simulink model "angularOnlinePIDTuningR2019a"  (R2019a)
settings: Solver=FixedStepAuto  StartTime=0.0  StopTime=100  RelTol=1e-3
model workspace (MAT data in the model file):
  p = [-7.82997288351e-05; 0.181210895977; -0.072497134344; 0.000486358314052; 0.0361674637937]
libraries: arduinolib x7, simulink x3, slctrlblks x1, simulink_extras x1
settings Model: SimulationMode=external  ExtModeTrigDuration=2  Creator=The MathWorks, Inc.  LastModifiedBy=manh
settings DataIOCC: ReturnWorkspaceOutputs=off
settings OptimizationCC: PassReuseOutputArgsAs=Individual arguments  MaxStackSize=64
settings DebuggingCC: ParameterPrecisionLossMsg=none  ParameterTunabilityLossMsg=error  ArithmeticOperatorsInVariantConditions=warning
settings HardwareCC: ProdBitPerInt=16  ProdBitPerPointer=16  ProdBitPerSizeT=16  ProdBitPerPtrDiffT=16  ProdLargestAtomicFloat=None  ProdWordSize=8  ProdHWDeviceType=Atmel->AVR
settings SFSimCC: SimUseLocalCustomCode=off  MATLABDynamicMemAlloc=off
settings RTWCC: SystemTargetFile=ert.tlc  HardwareBoard=Arduino Mega 2560  TLCOptions=-aInlineSetEventsForThisBaseRateFcn=TLC_FALSE -aSuppressMultiTaskScheduler=TLC_FALSE -aRateBasedStepFcn=1  TemplateMakefile=ert_default_tmf  GenerateReport=on  RTWUseLocalCustomCode=off  Toolchain=Arduino AVR  BuildConfiguration=Faster Runs  IncludeHyperlinkInReport=on  LaunchReport=on  GenerateTraceInfo=on  GenerateTraceReport=on  GenerateTraceReportSl=on  GenerateTraceReportSf=on  GenerateTraceReportEml=on
settings CodeAppCC: ForceParamTrailComments=on  IgnoreCustomStorageClasses=off  OperatorAnnotations=on  SimulinkDataObjDesc=on  SFDataObjDesc=on  InsertBlockDesc=on
settings ERTTargetCC: SupportContinuousTime=on  SupportVariableSizeSignals=on

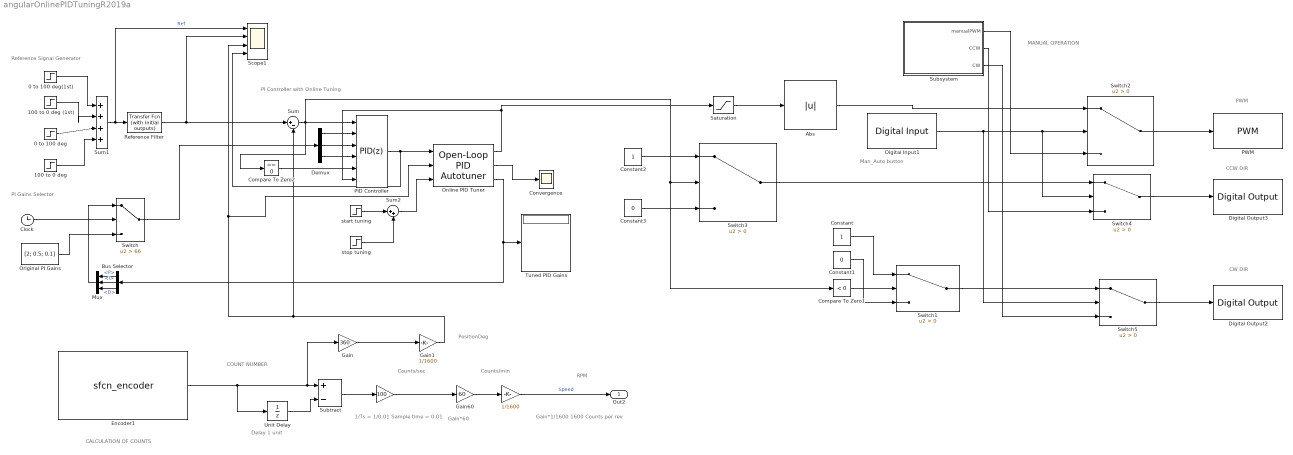
== system angularOnlinePIDTuningR2019a ==
  note: PI Gains Selector
  note: PI Controller with Online Tuning
  note: Reference Signal Generator
  note: COUNT NUMBER
  note: Gain*1/1600
      | 1600 Counts per rev
  note: Man_Auto button
  note: Counts/sec
  note: CW DIR
  note: CALCULATION OF COUNTS
  note: MANUAL OPERATION
  note: Delay 1 unit
  note: PWM
  note: Gain*60
  note: RPM
  note: Counts/min
  note: CCW DIR
  note: 1/Ts = 1/0.01
      | Sample time = 0.01
  note: PositionDeg
  " " : Gain  Gain=100  OutDataTypeStr=double
  " " : Gain  Gain=1/1600  OutDataTypeStr=double
  "0 to 100 deg " : Step  Time=60  After=100  SampleTime=0
  0 to 100 deg(1st) : Step  Time=2  After=100  SampleTime=0
  100 to 0 deg : Step  Time=80  After=-100  SampleTime=0
  100 to 0 deg (1st) : Step  Time=20  After=-100  SampleTime=0
  Abs : Abs
  Bus Selector : BusSelector  OutputSignals=P,I,D
  Clock : Clock
  Compare To Zero1 : simulink/Logic and Bit Operations/Compare To Zero  relop=<  OutDataTypeStr=boolean
  Compare To Zero2 : simulink/Logic and Bit Operations/Compare To Zero  relop===  OutDataTypeStr=boolean
  Constant : Constant
  Constant1 : Constant  Value=0
  Constant2 : Constant
  Constant3 : Constant  Value=0
  Convergence : Scope
  Demux : Demux  Outputs=3
  Digital Input1 : arduinolib/Digital Input  pinNumber=28  sampleTime=0.01  blockPlatform=arduino
      settings: SourceProductName=Simulink Support Package for Arduino Hardware
  Digital Output2 : arduinolib/Digital Output  pinNumber=38  blockPlatform=arduino
  Digital Output3 : arduinolib/Digital Output  pinNumber=36  blockPlatform=arduino
  Encoder1 : S-Function  InitFcn=try, set_param(gcb,'FunctionName','sfcn_encoder'), end  FunctionName=sfcn_encoder  Parameters=uint8(0),uint8(2),uint8(3)  SFunctionModules=sfcn_encoder_wrapper  SFunctionDeploymentMode=off  EnableBusSupport=off  mask(S-Function Builder){}
      mask init:
      | val = [[.9  0.75 0.75 1 1 .9 .9 1]',[1 1 0.75 0.75 .9 .9 1 .9]'];try , sys = get_param(gcb,'SfunBuilderFcnName');if isempty(sys), sys = get_param(gcb,'FunctionName'); end,catch, sys = get_param(gcb,'FunctionName'); end
      settings: CopyFcn=set_param(gcbh,'LinkStatus','none')  PreSaveFcn=try, set_param(gcb,'FunctionName','sfcn_encoder'), end  OpenFcn=sfunctionwizard(gcbh)
      mask Display: plot(val(:,1),val(:,2)),disp(sys), port_label('output',1,'pos')
  Gain : Gain  Gain=360  ParamDataTypeStr=double  OutDataTypeStr=double
  Gain1 : Gain  Gain=1/1600  ParamDataTypeStr=double  OutDataTypeStr=double
  Gain60 : Gain  Gain=60  OutDataTypeStr=double
  Mux : Mux  Inputs=3
  Online PID Tuner : slctrlblks/Open-Loop PID Autotuner  PIDType=PID  PIDForm=Parallel  TimeDomain=discrete-time  DiscreteTs=0.1  IntegratorFormula=Forward Euler  FilterFormula=Forward Euler  ContinuousTs=0.02  Bandwidth=2  UseExternalWC=off  TargetPM=60  UseExternalPM=off  UseExternalAchievedPM=off  AmpSine=0.1  UseExternalAmpSine=off  EstimateDCGain=on  AmpStep=0.1  UseExternalAmpStep=off  UseExternalFRD=off  UseExternalU0=off  UseExternalDCGain=off  NotDeployTuningModule=on  UsePLCCoder=off  BlockDataType=double  UseConnectedPID=on  blockpath=[]  tunedP=0  tunedI=0  tunedD=0  tunedN=100  tunedPM=0  EstimationWindowSize=4
      settings: SourceProductName=Simulink Control Design  SourceProductBaseCode=SD
  Original PI Gains : Constant  Value=[2; 0.5; 0.1]
  PID Controller : simulink/Continuous/PID Controller  Tag=PID1  Controller=PID  Form=Parallel  TimeDomain=Discrete-time  SampleTime=0.01  IntegratorMethod=Forward Euler  FilterMethod=Forward Euler  ControllerParametersSource=external  P=0.01  I=0.01  D=0  UseFilter=off  N=100  TunerSelectOption=Transfer Function Based (PID Tuner App)  ZeroCross=off  InitialConditionSource=internal  InitialConditionForIntegrator=0  InitialConditionForFilter=0  DifferentiatorICPrevScaledInput=0  ExternalReset=either  TrackingMode=on  Kt=1  LimitOutput=on  UpperSaturationLimit=255  LowerSaturationLimit=-255  LinearizeAsGain=off  AntiWindupMode=back-calculation  Kb=1  POutMin=[ ]  POutMax=[ ]  IOutMin=[ ]  IOutMax=[ ]  DOutMin=[ ]  DOutMax=[ ]  NOutMin=[ ]  NOutMax=[ ]  SumOutMin=[ ]  SumOutMax=[ ]  SaturationOutMin=[ ]  SaturationOutMax=[ ]  PParamMin=[ ]  PParamMax=[ ]  IParamMin=[ ]  IParamMax=[ ]  DParamMin=[ ]  DParamMax=[ ]  NParamMin=[ ]  NParamMax=[ ]  KbParamMin=[ ]  KbParamMax=[ ]  KtParamMin=[ ]  KtParamMax=[ ]  KbOutMin=[ ]  KbOutMax=[ ]  KtOutMin=[ ]  KtOutMax=[ ]  IntegratorOutMin=[ ]  IntegratorOutMax=[ ]  FilterOutMin=[ ]  FilterOutMax=[ ]  SumI1OutMin=[ ]  SumI1OutMax=[ ]  SumI2OutMin=[ ]  SumI2OutMax=[ ]  SumI3OutMin=[ ]  SumI3OutMax=[ ]  SumI4OutMin=[]  SumI4OutMax=[]  SumDOutMin=[ ]  SumDOutMax=[ ]  DifferentiatorOutMin=[]  DifferentiatorOutMax=[]  FilterDiffOutCoefMin=[]  FilterDiffOutCoefMax=[]  ReciprocalOutMin=[]  ReciprocalOutMax=[]  SumDenOutMin=[]  SumDenOutMax=[]  SumNumOutMin=[]  SumNumOutMax=[]  DivideOutMin=[]  DivideOutMax=[]  IntegratorContinuousStateAttributes=''  IntegratorStateMustResolveToSignalObject=off  IntegratorRTWStateStorageClass=Auto  FilterContinuousStateAttributes=''  FilterStateMustResolveToSignalObject=off  FilterRTWStateStorageClass=Auto  ParallelPVariant=ExternalParameters  IdealPVariant=Disabled  IVariant=ExternalParameters  DVariant=ExternalParameters  IntegratorVariant=Discrete  SatVariant=Enabled  AWVariant=BackCalculation  PCopyVariant=Disabled  TRVariant=Enabled  FdbkBlocksVariant=Forward  IdealPFdbkVariant=Disabled  SatFdbkVariant=Disabled  DerivativeFilterVariant=Differentiator  NVariant=Passthrough  NCopyVariant=Disabled_SignalSpec  FilterICVariant=InternalICsDifferentiator  IntegratorICVariant=InternalICs  ExternalResetVariant=ExternalReset  TRSumVariant=TrackingMode  SumFdbkVariant=Disabled  SumVariant=Sum_PID
  PWM : arduinolib/PWM  pinNumber=7  EnableInputFrequency=off  InitialFrequency=2000  InitialDutyCycle=0  NotificationType=None  blockPlatform=arduino
  Reference Filter : simulink_extras/Additional Linear/Transfer Fcn (with initial outputs)  N=[10]  D="[1  10]"  Y0=0  U0=0
  Saturation : Saturate  UpperLimit=255  LowerLimit=-255
  Scope1 : Scope  NumInputPorts=4
  Subsystem : Subsystem
  Subtract : Sum  Inputs=+-
  Sum : Sum  Inputs=|+-
  Sum1 : Sum  Inputs=|++++
  Sum2 : Sum  Inputs=|++
  Switch : Switch  Criteria=u2 > Threshold  Threshold=66
  Switch{1..5} (5 alike) : Switch  Criteria=u2 > Threshold
  Tuned PID Gains : Display
  Unit Delay : UnitDelay  SampleTime=-1  HasFrameUpgradeWarning=on
  start tuning : Step  Time=30  SampleTime=0
  stop tuning : Step  Time=65  After=-1  SampleTime=0
  Out2 : Outport  SignalName=speedRPM
  wires:
  Bus Selector/1 -> Mux/1  "<P>"
  100 to 0 deg/1 -> Sum1/4
  Original PI Gains/1 -> Switch/3
  Bus Selector/2 -> Mux/2  "<I>"
  Online PID Tuner/1 -> Saturation/1, PID Controller/6
  Online PID Tuner/3 -> Bus Selector/1, Tuned PID Gains/1
  Demux/1 -> PID Controller/2
  PID Controller/1 -> Scope1/4, Online PID Tuner/1
  Sum1/1 -> Scope1/1, Reference Filter/1  "Ref"
  Sum/1 -> Compare To Zero1/1, Switch3/2, PID Controller/1, Compare To Zero2/1
  Reference Filter/1 -> Sum/1, Scope1/2
  "0 to 100 deg "/1 -> Sum1/3
  Online PID Tuner/2 -> Convergence/1
  Demux/2 -> PID Controller/3
  Sum2/1 -> Online PID Tuner/3
  stop tuning/1 -> Sum2/2
  start tuning/1 -> Sum2/1
  100 to 0 deg (1st)/1 -> Sum1/2
  Switch/1 -> Demux/1
  Mux/1 -> Switch/1
  Gain1/1 -> Sum/2, Online PID Tuner/2, Scope1/3
  Switch3/1 -> Switch4/1
  " "/1 -> Out2/1  "Speed"
  Subsystem/2(CCW) -> Switch4/3
  Gain60/1 -> " "/1
  Gain/1 -> Gain1/1
  Switch2/1 -> PWM/1
  Switch1/1 -> Switch5/1
  Subsystem/3(CW) -> Switch5/3
  Constant/1 -> Switch1/1
  Saturation/1 -> Abs/1
  Abs/1 -> Switch2/1
  Constant1/1 -> Switch1/3
  Constant3/1 -> Switch3/3
  Constant2/1 -> Switch3/1
  " "/1 -> Gain60/1
  Unit Delay/1 -> Subtract/2
  Subsystem/1(manualPWM) -> Switch2/3
  Encoder1/1 -> Gain/1, Subtract/1, Unit Delay/1
  Switch4/1 -> Digital Output3/1
  Switch5/1 -> Digital Output2/1
  Subtract/1 -> " "/1
  Digital Input1/1 -> Switch2/2, Switch4/2, Switch5/2
  Clock/1 -> Switch/2
  0 to 100 deg(1st)/1 -> Sum1/1
  Compare To Zero1/1 -> Switch1/2
  Bus Selector/3 -> Mux/3  "<D>"
  Compare To Zero2/1 -> PID Controller/5
  Demux/3 -> PID Controller/4

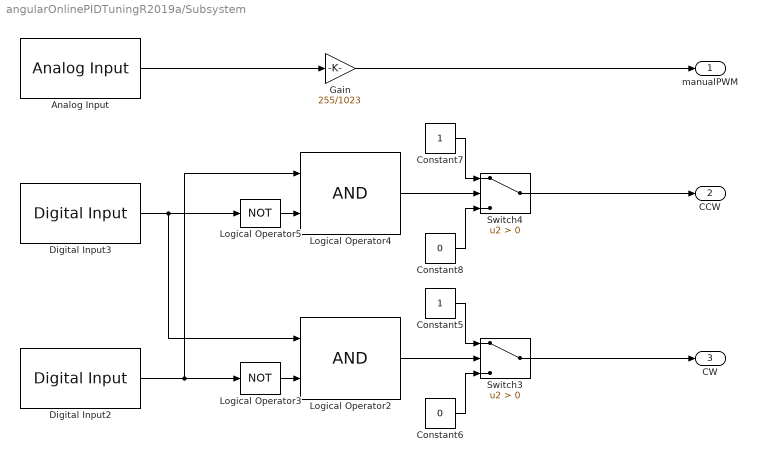
== system angularOnlinePIDTuningR2019a/Subsystem ==
  Analog Input : arduinolib/Analog Input  pinNumber=5  sampleTime=0.01  blockPlatform=arduino
  Constant5 : Constant
  Constant6 : Constant  Value=0
  Constant7 : Constant
  Constant8 : Constant  Value=0
  Digital Input2 : arduinolib/Digital Input  pinNumber=22  sampleTime=0.01  blockPlatform=arduino
      settings: SourceProductName=Simulink Support Package for Arduino Hardware
  Digital Input3 : arduinolib/Digital Input  pinNumber=24  sampleTime=0.01  blockPlatform=arduino
      settings: SourceProductName=Simulink Support Package for Arduino Hardware
  Gain : Gain  Gain=255/1023
  Logical Operator2 : Logic  AllPortsSameDT=off  OutDataTypeStr=boolean
  Logical Operator3 : Logic  Operator=NOT  AllPortsSameDT=off  OutDataTypeStr=boolean
  Logical Operator4 : Logic  AllPortsSameDT=off  OutDataTypeStr=boolean
  Logical Operator5 : Logic  Operator=NOT  AllPortsSameDT=off  OutDataTypeStr=boolean
  Switch3 : Switch  Criteria=u2 > Threshold
  Switch4 : Switch  Criteria=u2 > Threshold
  manualPWM : Outport
  CCW : Outport  Port=2
  CW : Outport  Port=3
  wires:
  Constant6/1 -> Switch3/3
  Constant7/1 -> Switch4/1
  Logical Operator5/1 -> Logical Operator4/2
  Constant5/1 -> Switch3/1
  Switch3/1 -> CW/1
  Logical Operator3/1 -> Logical Operator2/2
  Logical Operator2/1 -> Switch3/2
  Switch4/1 -> CCW/1
  Digital Input2/1 -> Logical Operator4/1, Logical Operator3/1
  Gain/1 -> manualPWM/1
  Analog Input/1 -> Gain/1
  Logical Operator4/1 -> Switch4/2
  Digital Input3/1 -> Logical Operator5/1, Logical Operator2/1
  Constant8/1 -> Switch4/3
